simulink subsystem "controller_lqr_only"  (R2025b)
settings: Solver=VariableStepAuto  StartTime=0.0  StopTime=10.0  RelTol=1e-3
undefined symbols (not defined in the file or in its folder): dt_data
settings Model: Creator=koryh  LastModifiedBy=kjhaydon

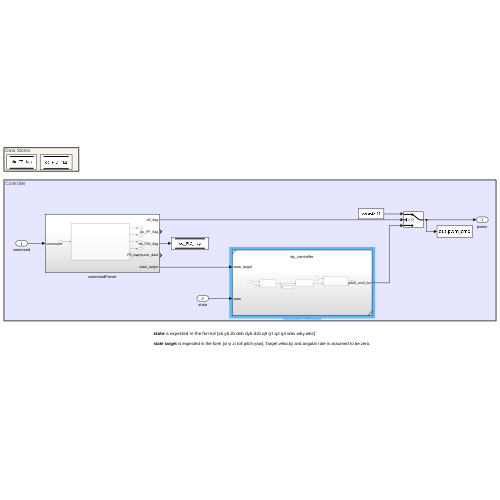
[thumbnail: Simulink's stored preview of the top-level diagram]
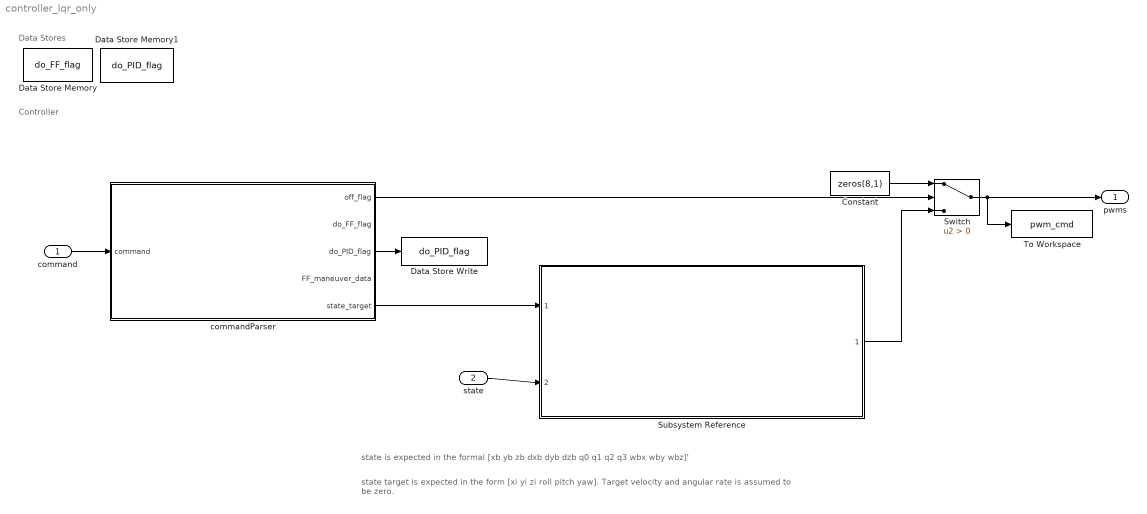
== system controller_lqr_only ==
  note: state target is expected in the form [xi yi zi roll pitch yaw]. Target velocity and angular rate is assumed to be zero.
  note: Controller
  note: Data Stores
  note: state is expected in the formal [xb yb zb dxb dyb dzb q0 q1 q2 q3 wbx wby wbz]'
  command : Inport
  state : Inport  Port=2
  Constant : Constant  Value=zeros(8,1)
  Data Store Memory : DataStoreMemory  DataStoreName=do_FF_flag  WriteAfterWriteMsg=warning  ShowAdditionalParam=off
  Data Store Memory1 : DataStoreMemory  DataStoreName=do_PID_flag  WriteAfterWriteMsg=warning  ShowAdditionalParam=off
  Data Store Write : DataStoreWrite  DataStoreName=do_PID_flag  IndexOptions=Index vector (dialog)  Indices=1  OutputSizes=1
  Subsystem Reference : Subsystem  ReferencedSubsystem=lqr_controller
  Switch : Switch  Criteria=u2 > Threshold  SaturateOnIntegerOverflow=off  InputSameDT=off
  To Workspace : ToWorkspace  VariableName=pwm_cmd  SaveFormat=Timeseries  SampleTime=dt_data
  commandParser : Subsystem
  pwms : Outport
  wires:
  command/1 -> commandParser/1(command)
  Switch/1 -> To Workspace/1, pwms/1
  commandParser/1(off_flag) -> Switch/2
  Constant/1 -> Switch/1
  commandParser/3(do_PID_flag) -> Data Store Write/1
  commandParser/5(state_target) -> Subsystem Reference/1
  state/1 -> Subsystem Reference/2
  Subsystem Reference/1 -> Switch/3

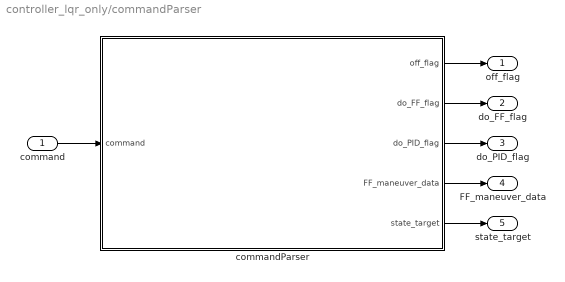
== system controller_lqr_only/commandParser ==
  command : Inport
  commandParser : MATLAB Function  TreatAsAtomicUnit=on
  off_flag : Outport
  do_FF_flag : Outport  Port=2
  do_PID_flag : Outport  Port=3
  FF_maneuver_data : Outport  Port=4
  state_target : Outport  Port=5
  wires:
  commandParser/1(off_flag) -> off_flag/1
  commandParser/2(do_FF_flag) -> do_FF_flag/1
  commandParser/5(state_target) -> state_target/1
  commandParser/4(FF_maneuver_data) -> FF_maneuver_data/1
  commandParser/3(do_PID_flag) -> do_PID_flag/1
  command/1 -> commandParser/1(command)

== matlab function controller_lqr_only/commandParser/commandParser ==
  data: command input; off_flag output; do_FF_flag output; do_PID_flag output; FF_maneuver_data output; state_target output
function [off_flag, do_FF_flag,do_PID_flag,FF_maneuver_data,state_target]    = fcn(command)

[off_flag, do_FF_flag,do_PID_flag,FF_maneuver_data,state_target] = commandParser(command);
